simulink model "Crazyflie_Position_controller"  (R2020b)
settings: Solver=VariableStepAuto  StartTime=0.0  StopTime=10.0  RelTol=1e-3
libraries: pid_lib x4
settings Model: Creator=kt012  LastModifiedBy=kt012

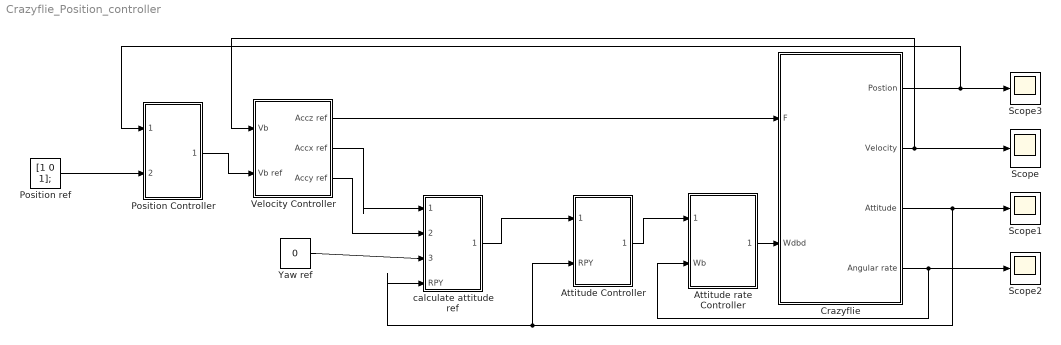
== system Crazyflie_Position_controller ==
  Attitude Controller : Subsystem
  Attitude rate Controller : Subsystem
  Crazyflie : Subsystem
  Position Controller : Subsystem
  Position ref : Constant  Value=[1 0 1];
  Scope{,1..3} (4 alike) : Scope
  Velocity Controller : Subsystem
  Yaw ref : Constant  Value=0
  calculate attitude ref : Subsystem
  wires:
  Crazyflie/1(Postion) -> Position Controller/1(Position), Scope3/1
  Crazyflie/2(Velocity) -> Velocity Controller/1(Vb), Scope/1
  Crazyflie/3(Attitude) -> Attitude Controller/2(RPY), calculate attitude ref/4(RPY), Scope1/1
  Crazyflie/4(Angular rate) -> Attitude rate Controller/2(Wb), Scope2/1
  Attitude rate Controller/1(Wdb_ref) -> Crazyflie/2(Wdbd)
  Attitude Controller/1(Wb_ref) -> Attitude rate Controller/1(Wb_ref)
  Velocity Controller/1(Accz ref) -> Crazyflie/1(F)
  Position Controller/1(Vel ref) -> Velocity Controller/2(Vb ref)
  Velocity Controller/2(Accx ref) -> calculate attitude ref/1(Accel x)
  Velocity Controller/3(Accy ref) -> calculate attitude ref/2("Accel y ")
  Yaw ref/1 -> calculate attitude ref/3(Yaw ref)
  calculate attitude ref/1(Attitude ref) -> Attitude Controller/1(RPY_ref)
  Position ref/1 -> Position Controller/2(Position ref)

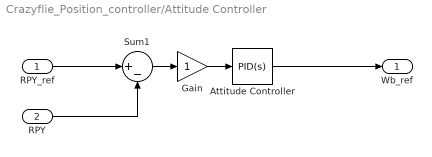
== system Crazyflie_Position_controller/Attitude Controller ==
  RPY_ref : Inport
  RPY : Inport  Port=2
  Attitude Controller : pid_lib/PID Controller  Controller=PID  Form=Parallel  TimeDomain=Continuous-time  UseExternalTs=off  SampleTime=-1  IntegratorMethod=Forward Euler  FilterMethod=Forward Euler  ControllerParametersSource=internal  P=6.0 * 180 / 3.14  I=3.0 * 180 / 3.14  D=25  UseFilter=on  N=100  TunerSelectOption=Transfer Function Based (PID Tuner App)  InitialConditionSource=internal  InitialConditionForIntegrator=0  InitialConditionForFilter=0  DifferentiatorICPrevScaledInput=0  ExternalReset=none  TrackingMode=off  Kt=1  LimitOutput=off  SatLimitsSource=internal  UpperSaturationLimit=inf  LowerSaturationLimit=-inf  LinearizeAsGain=on  AntiWindupMode=none  Kb=1  POutMin=[]  POutMax=[]  IOutMin=[]  IOutMax=[]  DOutMin=[]  DOutMax=[]  NOutMin=[]  NOutMax=[]  SumOutMin=[]  SumOutMax=[]  SaturationOutMin=[]  SaturationOutMax=[]  PParamMin=[]  PParamMax=[]  IParamMin=[]  IParamMax=[]  DParamMin=[]  DParamMax=[]  NParamMin=[]  NParamMax=[]  KbParamMin=[]  KbParamMax=[]  KtParamMin=[]  KtParamMax=[]  KbOutMin=[]  KbOutMax=[]  KtOutMin=[]  KtOutMax=[]  IntegratorOutMin=[]  IntegratorOutMax=[]  FilterOutMin=[]  FilterOutMax=[]  SumI1OutMin=[]  SumI1OutMax=[]  SumI2OutMin=[]  SumI2OutMax=[]  SumI3OutMin=[]  SumI3OutMax=[]  SumI4OutMin=[]  SumI4OutMax=[]  SumDOutMin=[]  SumDOutMax=[]  DifferentiatorOutMin=[]  DifferentiatorOutMax=[]  FilterDiffOutCoefMin=[]  FilterDiffOutCoefMax=[]  ReciprocalOutMin=[]  ReciprocalOutMax=[]  SumDenOutMin=[]  SumDenOutMax=[]  SumNumOutMin=[]  SumNumOutMax=[]  DivideOutMin=[]  DivideOutMax=[]  UdiffTsProdOutMin=[]  UdiffTsProdOutMax=[]  NTsProdOutMin=[]  NTsProdOutMax=[]  UintegralTsProdOutMin=[]  UintegralTsProdOutMax=[]  UngainTsProdOutMin=[]  UngainTsProdOutMax=[]  IntegratorContinuousStateAttributes=''  IntegratorStateMustResolveToSignalObject=off  IntegratorRTWStateStorageClass=Auto  FilterContinuousStateAttributes=''  FilterStateMustResolveToSignalObject=off  FilterRTWStateStorageClass=Auto  ParallelPVariant=InternalParameters  IdealPVariant=Disabled  IVariant=InternalParameters  DVariant=InternalParameters  IntegratorVariant=Continuous  SatVariant=Disabled  AWVariant=Passthrough  PCopyVariant=Disabled  TRVariant=Disabled  FdbkBlocksVariant=Forward  IdealPFdbkVariant=Disabled  SatFdbkVariant=Disabled  DerivativeFilterVariant=ContFilter  NVariant=InternalParameters  NCopyVariant=Disabled  FilterICVariant=InternalICsFilter  IntegratorICVariant=InternalICs  ExternalResetVariant=Disabled  TRSumVariant=Passthrough  SumFdbkVariant=Disabled  SumVariant=Sum_PID  TsampFilterVariant=InternalTs  TsampNgainVariant=Passthrough  TsampIntegralVariant=Passthrough  ExternalSaturationOutDataTypeStr=Inherit: Same as second input
  Gain : Gain
  Sum1 : Sum  Inputs=|+-
  Wb_ref : Outport
  wires:
  Gain/1 -> Attitude Controller/1
  RPY/1 -> Sum1/2
  Sum1/1 -> Gain/1
  Attitude Controller/1 -> Wb_ref/1
  RPY_ref/1 -> Sum1/1

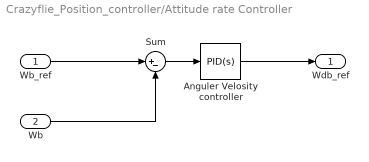
== system Crazyflie_Position_controller/Attitude rate Controller ==
  Wb_ref : Inport
  Wb : Inport  Port=2
  Anguler Velosity controller : pid_lib/PID Controller  Controller=PID  Form=Parallel  TimeDomain=Continuous-time  UseExternalTs=off  SampleTime=-1  IntegratorMethod=Forward Euler  FilterMethod=Forward Euler  ControllerParametersSource=internal  P=250 * 180 / 3.14  I=500 * 180 / 3.14  D=2.5 * 180 / 3.14  UseFilter=on  N=100  TunerSelectOption=Transfer Function Based (PID Tuner App)  InitialConditionSource=internal  InitialConditionForIntegrator=0  InitialConditionForFilter=0  DifferentiatorICPrevScaledInput=0  ExternalReset=none  TrackingMode=off  Kt=1  LimitOutput=off  SatLimitsSource=internal  UpperSaturationLimit=inf  LowerSaturationLimit=-inf  LinearizeAsGain=on  AntiWindupMode=none  Kb=1  POutMin=[]  POutMax=[]  IOutMin=[]  IOutMax=[]  DOutMin=[]  DOutMax=[]  NOutMin=[]  NOutMax=[]  SumOutMin=[]  SumOutMax=[]  SaturationOutMin=[]  SaturationOutMax=[]  PParamMin=[]  PParamMax=[]  IParamMin=[]  IParamMax=[]  DParamMin=[]  DParamMax=[]  NParamMin=[]  NParamMax=[]  KbParamMin=[]  KbParamMax=[]  KtParamMin=[]  KtParamMax=[]  KbOutMin=[]  KbOutMax=[]  KtOutMin=[]  KtOutMax=[]  IntegratorOutMin=[]  IntegratorOutMax=[]  FilterOutMin=[]  FilterOutMax=[]  SumI1OutMin=[]  SumI1OutMax=[]  SumI2OutMin=[]  SumI2OutMax=[]  SumI3OutMin=[]  SumI3OutMax=[]  SumI4OutMin=[]  SumI4OutMax=[]  SumDOutMin=[]  SumDOutMax=[]  DifferentiatorOutMin=[]  DifferentiatorOutMax=[]  FilterDiffOutCoefMin=[]  FilterDiffOutCoefMax=[]  ReciprocalOutMin=[]  ReciprocalOutMax=[]  SumDenOutMin=[]  SumDenOutMax=[]  SumNumOutMin=[]  SumNumOutMax=[]  DivideOutMin=[]  DivideOutMax=[]  UdiffTsProdOutMin=[]  UdiffTsProdOutMax=[]  NTsProdOutMin=[]  NTsProdOutMax=[]  UintegralTsProdOutMin=[]  UintegralTsProdOutMax=[]  UngainTsProdOutMin=[]  UngainTsProdOutMax=[]  IntegratorContinuousStateAttributes=''  IntegratorStateMustResolveToSignalObject=off  IntegratorRTWStateStorageClass=Auto  FilterContinuousStateAttributes=''  FilterStateMustResolveToSignalObject=off  FilterRTWStateStorageClass=Auto  ParallelPVariant=InternalParameters  IdealPVariant=Disabled  IVariant=InternalParameters  DVariant=InternalParameters  IntegratorVariant=Continuous  SatVariant=Disabled  AWVariant=Passthrough  PCopyVariant=Disabled  TRVariant=Disabled  FdbkBlocksVariant=Forward  IdealPFdbkVariant=Disabled  SatFdbkVariant=Disabled  DerivativeFilterVariant=ContFilter  NVariant=InternalParameters  NCopyVariant=Disabled  FilterICVariant=InternalICsFilter  IntegratorICVariant=InternalICs  ExternalResetVariant=Disabled  TRSumVariant=Passthrough  SumFdbkVariant=Disabled  SumVariant=Sum_PID  TsampFilterVariant=InternalTs  TsampNgainVariant=Passthrough  TsampIntegralVariant=Passthrough  ExternalSaturationOutDataTypeStr=Inherit: Same as second input
  Sum : Sum  Inputs=|+-
  Wdb_ref : Outport
  wires:
  Sum/1 -> Anguler Velosity controller/1
  Anguler Velosity controller/1 -> Wdb_ref/1
  Wb/1 -> Sum/2
  Wb_ref/1 -> Sum/1

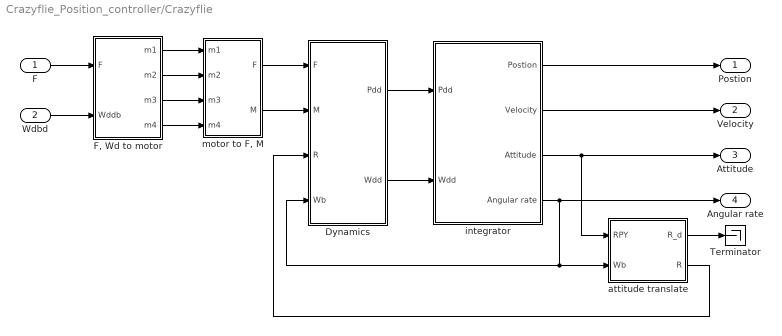
== system Crazyflie_Position_controller/Crazyflie ==
  F : Inport
  Wdbd : Inport  Port=2
  Dynamics : MATLAB Function  TreatAsAtomicUnit=on
  "F, Wd to motor" : MATLAB Function  TreatAsAtomicUnit=on
  Terminator : Terminator
  attitude translate : MATLAB Function  TreatAsAtomicUnit=on
  integrator : Subsystem
  "motor to F, M" : MATLAB Function  TreatAsAtomicUnit=on
  Postion : Outport
  Velocity : Outport  Port=2
  Attitude : Outport  Port=3
  Angular rate : Outport  Port=4
  wires:
  "F, Wd to motor"/1(m1) -> "motor to F, M"/1(m1)
  Wdbd/1 -> "F, Wd to motor"/2(Wddb)
  "F, Wd to motor"/4(m4) -> "motor to F, M"/4(m4)
  "F, Wd to motor"/2(m2) -> "motor to F, M"/2(m2)
  "F, Wd to motor"/3(m3) -> "motor to F, M"/3(m3)
  Dynamics/2(Wdd) -> integrator/2(Wdd)
  "motor to F, M"/2(M) -> Dynamics/2(M)
  integrator/4(Angular rate) -> Angular rate/1, attitude translate/2(Wb), Dynamics/4(Wb)
  "motor to F, M"/1(F) -> Dynamics/1(F)
  F/1 -> "F, Wd to motor"/1(F)
  Dynamics/1(Pdd) -> integrator/1(Pdd)
  integrator/3(Attitude) -> Attitude/1, attitude translate/1(RPY)
  integrator/1(Postion) -> Postion/1
  integrator/2(Velocity) -> Velocity/1
  attitude translate/2(R) -> Dynamics/3(R)
  attitude translate/1(R_d) -> Terminator/1

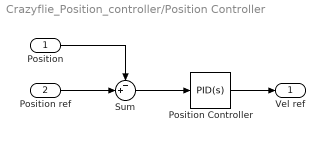
== system Crazyflie_Position_controller/Position Controller ==
  Position : Inport
  Position ref : Inport  Port=2
  Position Controller : pid_lib/PID Controller  Controller=PID  Form=Parallel  TimeDomain=Continuous-time  UseExternalTs=off  SampleTime=-1  IntegratorMethod=Forward Euler  FilterMethod=Forward Euler  ControllerParametersSource=internal  P=2  I=0.5  D=0  UseFilter=on  N=100  TunerSelectOption=Transfer Function Based (PID Tuner App)  InitialConditionSource=internal  InitialConditionForIntegrator=0  InitialConditionForFilter=0  DifferentiatorICPrevScaledInput=0  ExternalReset=none  TrackingMode=off  Kt=1  LimitOutput=off  SatLimitsSource=internal  UpperSaturationLimit=inf  LowerSaturationLimit=-inf  LinearizeAsGain=on  AntiWindupMode=none  Kb=1  POutMin=[]  POutMax=[]  IOutMin=[]  IOutMax=[]  DOutMin=[]  DOutMax=[]  NOutMin=[]  NOutMax=[]  SumOutMin=[]  SumOutMax=[]  SaturationOutMin=[]  SaturationOutMax=[]  PParamMin=[]  PParamMax=[]  IParamMin=[]  IParamMax=[]  DParamMin=[]  DParamMax=[]  NParamMin=[]  NParamMax=[]  KbParamMin=[]  KbParamMax=[]  KtParamMin=[]  KtParamMax=[]  KbOutMin=[]  KbOutMax=[]  KtOutMin=[]  KtOutMax=[]  IntegratorOutMin=[]  IntegratorOutMax=[]  FilterOutMin=[]  FilterOutMax=[]  SumI1OutMin=[]  SumI1OutMax=[]  SumI2OutMin=[]  SumI2OutMax=[]  SumI3OutMin=[]  SumI3OutMax=[]  SumI4OutMin=[]  SumI4OutMax=[]  SumDOutMin=[]  SumDOutMax=[]  DifferentiatorOutMin=[]  DifferentiatorOutMax=[]  FilterDiffOutCoefMin=[]  FilterDiffOutCoefMax=[]  ReciprocalOutMin=[]  ReciprocalOutMax=[]  SumDenOutMin=[]  SumDenOutMax=[]  SumNumOutMin=[]  SumNumOutMax=[]  DivideOutMin=[]  DivideOutMax=[]  UdiffTsProdOutMin=[]  UdiffTsProdOutMax=[]  NTsProdOutMin=[]  NTsProdOutMax=[]  UintegralTsProdOutMin=[]  UintegralTsProdOutMax=[]  UngainTsProdOutMin=[]  UngainTsProdOutMax=[]  IntegratorContinuousStateAttributes=''  IntegratorStateMustResolveToSignalObject=off  IntegratorRTWStateStorageClass=Auto  FilterContinuousStateAttributes=''  FilterStateMustResolveToSignalObject=off  FilterRTWStateStorageClass=Auto  ParallelPVariant=InternalParameters  IdealPVariant=Disabled  IVariant=InternalParameters  DVariant=InternalParameters  IntegratorVariant=Continuous  SatVariant=Disabled  AWVariant=Passthrough  PCopyVariant=Disabled  TRVariant=Disabled  FdbkBlocksVariant=Forward  IdealPFdbkVariant=Disabled  SatFdbkVariant=Disabled  DerivativeFilterVariant=ContFilter  NVariant=InternalParameters  NCopyVariant=Disabled  FilterICVariant=InternalICsFilter  IntegratorICVariant=InternalICs  ExternalResetVariant=Disabled  TRSumVariant=Passthrough  SumFdbkVariant=Disabled  SumVariant=Sum_PID  TsampFilterVariant=InternalTs  TsampNgainVariant=Passthrough  TsampIntegralVariant=Passthrough  ExternalSaturationOutDataTypeStr=Inherit: Same as second input
  Sum : Sum  Inputs=-+|
  Vel ref : Outport
  wires:
  Sum/1 -> Position Controller/1
  Position Controller/1 -> Vel ref/1
  Position ref/1 -> Sum/2
  Position/1 -> Sum/1

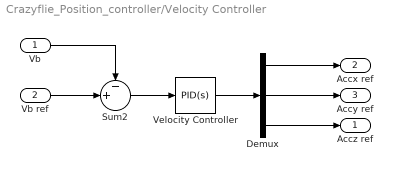
== system Crazyflie_Position_controller/Velocity Controller ==
  Vb : Inport
  Vb ref : Inport  Port=2
  Demux : Demux  Outputs=3
  Sum2 : Sum  Inputs=-+|
  Velocity Controller : pid_lib/PID Controller  Controller=PID  Form=Parallel  TimeDomain=Continuous-time  UseExternalTs=off  SampleTime=-1  IntegratorMethod=Forward Euler  FilterMethod=Forward Euler  ControllerParametersSource=internal  P=25  I=10  D=0  UseFilter=on  N=100  TunerSelectOption=Transfer Function Based (PID Tuner App)  InitialConditionSource=internal  InitialConditionForIntegrator=0  InitialConditionForFilter=0  DifferentiatorICPrevScaledInput=0  ExternalReset=none  TrackingMode=off  Kt=1  LimitOutput=off  SatLimitsSource=internal  UpperSaturationLimit=inf  LowerSaturationLimit=-inf  LinearizeAsGain=on  AntiWindupMode=none  Kb=1  POutMin=[]  POutMax=[]  IOutMin=[]  IOutMax=[]  DOutMin=[]  DOutMax=[]  NOutMin=[]  NOutMax=[]  SumOutMin=[]  SumOutMax=[]  SaturationOutMin=[]  SaturationOutMax=[]  PParamMin=[]  PParamMax=[]  IParamMin=[]  IParamMax=[]  DParamMin=[]  DParamMax=[]  NParamMin=[]  NParamMax=[]  KbParamMin=[]  KbParamMax=[]  KtParamMin=[]  KtParamMax=[]  KbOutMin=[]  KbOutMax=[]  KtOutMin=[]  KtOutMax=[]  IntegratorOutMin=[]  IntegratorOutMax=[]  FilterOutMin=[]  FilterOutMax=[]  SumI1OutMin=[]  SumI1OutMax=[]  SumI2OutMin=[]  SumI2OutMax=[]  SumI3OutMin=[]  SumI3OutMax=[]  SumI4OutMin=[]  SumI4OutMax=[]  SumDOutMin=[]  SumDOutMax=[]  DifferentiatorOutMin=[]  DifferentiatorOutMax=[]  FilterDiffOutCoefMin=[]  FilterDiffOutCoefMax=[]  ReciprocalOutMin=[]  ReciprocalOutMax=[]  SumDenOutMin=[]  SumDenOutMax=[]  SumNumOutMin=[]  SumNumOutMax=[]  DivideOutMin=[]  DivideOutMax=[]  UdiffTsProdOutMin=[]  UdiffTsProdOutMax=[]  NTsProdOutMin=[]  NTsProdOutMax=[]  UintegralTsProdOutMin=[]  UintegralTsProdOutMax=[]  UngainTsProdOutMin=[]  UngainTsProdOutMax=[]  IntegratorContinuousStateAttributes=''  IntegratorStateMustResolveToSignalObject=off  IntegratorRTWStateStorageClass=Auto  FilterContinuousStateAttributes=''  FilterStateMustResolveToSignalObject=off  FilterRTWStateStorageClass=Auto  ParallelPVariant=InternalParameters  IdealPVariant=Disabled  IVariant=InternalParameters  DVariant=InternalParameters  IntegratorVariant=Continuous  SatVariant=Disabled  AWVariant=Passthrough  PCopyVariant=Disabled  TRVariant=Disabled  FdbkBlocksVariant=Forward  IdealPFdbkVariant=Disabled  SatFdbkVariant=Disabled  DerivativeFilterVariant=ContFilter  NVariant=InternalParameters  NCopyVariant=Disabled  FilterICVariant=InternalICsFilter  IntegratorICVariant=InternalICs  ExternalResetVariant=Disabled  TRSumVariant=Passthrough  SumFdbkVariant=Disabled  SumVariant=Sum_PID  TsampFilterVariant=InternalTs  TsampNgainVariant=Passthrough  TsampIntegralVariant=Passthrough  ExternalSaturationOutDataTypeStr=Inherit: Same as second input
  Accz ref : Outport
  Accx ref : Outport  Port=2
  Accy ref : Outport  Port=3
  wires:
  Demux/2 -> Accy ref/1
  Velocity Controller/1 -> Demux/1
  Sum2/1 -> Velocity Controller/1
  Demux/1 -> Accx ref/1
  Vb/1 -> Sum2/1
  Demux/3 -> Accz ref/1
  Vb ref/1 -> Sum2/2

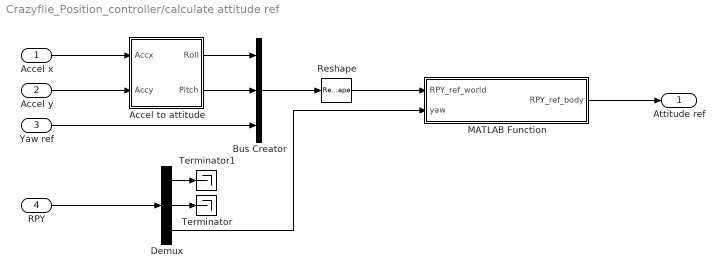
== system Crazyflie_Position_controller/calculate attitude ref ==
  Accel x : Inport
  "Accel y " : Inport  Port=2
  Yaw ref : Inport  Port=3
  RPY : Inport  Port=4
  Accel to attitude : MATLAB Function  TreatAsAtomicUnit=on
  Bus Creator : BusCreator  Inputs=3
  Demux : Demux  Outputs=3
  MATLAB Function : MATLAB Function  TreatAsAtomicUnit=on
  Reshape : Reshape  OutputDimensionality=Row vector (2-D)
  Terminator : Terminator
  Terminator1 : Terminator
  Attitude ref : Outport
  wires:
  Accel x/1 -> Accel to attitude/1(Accx)
  Accel to attitude/1(Roll) -> Bus Creator/1
  "Accel y "/1 -> Accel to attitude/2(Accy)
  Accel to attitude/2(Pitch) -> Bus Creator/2
  Yaw ref/1 -> Bus Creator/3
  MATLAB Function/1(RPY_ref_body) -> Attitude ref/1
  RPY/1 -> Demux/1
  Demux/3 -> MATLAB Function/2(yaw)
  Demux/2 -> Terminator/1
  Demux/1 -> Terminator1/1
  Reshape/1 -> MATLAB Function/1(RPY_ref_world)
  Bus Creator/1 -> Reshape/1

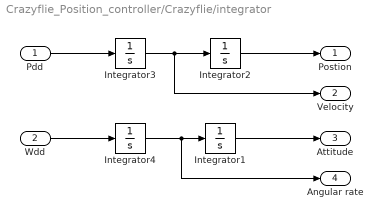
== system Crazyflie_Position_controller/Crazyflie/integrator ==
  Pdd : Inport
  Wdd : Inport  Port=2
  Integrator1 : Integrator  InitialCondition=[0 0 1];
  Integrator2 : Integrator  InitialCondition=[0 0 0];
  Integrator3 : Integrator  InitialCondition=[0 0 0];
  Integrator4 : Integrator  InitialCondition=[0 0 0];
  Postion : Outport
  Velocity : Outport  Port=2
  Attitude : Outport  Port=3
  Angular rate : Outport  Port=4
  wires:
  Wdd/1 -> Integrator4/1
  Integrator4/1 -> Angular rate/1, Integrator1/1
  Integrator1/1 -> Attitude/1
  Pdd/1 -> Integrator3/1
  Integrator3/1 -> Integrator2/1, Velocity/1
  Integrator2/1 -> Postion/1

== matlab function Crazyflie_Position_controller/Crazyflie/F, Wd to motor ==
  data: F input; Wddb input; m1 output; m2 output; m3 output; m4 output
 function [m1, m2, m3, m4]= fcn(F, Wddb)

% F [16bit] Wddb [16bit]
F = F * 1000 + 32000;

r = min(max(-32000, Wddb(1)), 32000)/2;
p = min(max(-32000, Wddb(2)), 32000)/2;
y = min(max(-32000, Wddb(3)), 32000);

m1 = min(max(0,F - r - p + y), 2^16);
m2 = min(max(0,F - r + p - y), 2^16);
m3 = min(max(0,F + r + p + y), 2^16);
m4 = min(max(0,F + r - p - y), 2^16);

% formation +
% r = min(max(-32000, Wddb(1)), 32000);
% p = min(max(-32000, Wddb(2)), 32000);
% y = min(max(-32000, Wddb(3)), 32000);
% m1 = min(max(0, + p + y), 2^16);
% m2 = min(max(0, - r - y), 2^16);
% m3 = min(max(0, - p + y), 2^16);
% m4 = min(max(0, + r - y), 2^16);

%         ^y
%         |
%         |
%   m3          m4
%
%                    ------>x
%
%   m2          m1

== matlab function Crazyflie_Position_controller/Crazyflie/attitude translate ==
  data: RPY input; Wb input; R_d output; R output
function [R_d, R]= fcn(RPY, Wb)
% 角速度 Vee演算
Wb = [ 0     -Wb(3)   Wb(2);
       Wb(3)  0       -Wb(1);
      -Wb(2)  Wb(1)   0   ];

% RPYから回転行列計算
roll = RPY(1);
pitch= RPY(2);
yaw = RPY(3);

R3 = [ cos(yaw) -sin(yaw) 0; sin(yaw) cos(yaw) 0; 0 0 1];              % ヨー角
R2 = [ cos(pitch) 0 -sin(pitch); 0 1 0; sin(pitch) 0 cos(pitch) ];     % ピッチ角
R1 = [ 1 0 0; 0 cos(roll) -sin(roll); 0 sin(roll) cos(roll)];          % ロール角

R = R1 * R2 * R3;   % 回転行列（ボディー　-> ワールド）

R_d = R * Wb;       % 微小時間の回転行列

== matlab function Crazyflie_Position_controller/calculate attitude ref/Accel to attitude ==
  data: Accx input; Roll output; Pitch output; Accy input
function [Roll, Pitch]= fcn(Accx, Accy)

Roll = -Accy * 3.14 / 180;
Pitch = -Accx* 3.14 / 180;

== matlab function Crazyflie_Position_controller/Crazyflie/motor to F, M ==
  data: F output; m1 input; m2 input; M output; m3 input; m4 input
function [F, M] = func(m1, m2, m3, m4)

% F [16bit] Wddb [16bit]

Armlength = 0.092/2;
m1 = 2.130295 * 10^(-11) * m1^2 + 1.032633 * 10^(-6) * m1 + 5.484560 * 10^(-4);
m2 = 2.130295 * 10^(-11) * m2^2 + 1.032633 * 10^(-6) * m2 + 5.484560 * 10^(-4);
m3 = 2.130295 * 10^(-11) * m3^2 + 1.032633 * 10^(-6) * m3 + 5.484560 * 10^(-4);
m4 = 2.130295 * 10^(-11) * m4^2 + 1.032633 * 10^(-6) * m4 + 5.484560 * 10^(-4);

% calculate thrust
F = m1 + m2 + m3 + m4;

% calculate moment formation X
M1 = Armlength / sqrt(2) * (m3 + m4 - m1 - m2);
M2 = -Armlength / sqrt(2) * (-m3 - m2 + m1 + m4);

% calculate moment formation + 
% M1 = Armlength  * (m4 - m2);
% M2 = Armlength * (m1 - m3);

M3 = m1 + m3 - m2 - m4;

M = [M1 M2 M3]';

== matlab function Crazyflie_Position_controller/Crazyflie/Dynamics ==
  data: Pdd output; F input; M input; R input; Wb input; Wdd output
function [Pdd,Wdd] = fcn(F, M, R, Wb)
m = 0.028;
e3 = [0 0 1]';
g = 9.8;
% % crazyflie
I = [16.571710 0.830806 0.718277;
     0.830806 16.655602 1.800197;
     0.718277 1.800197 29.261652] * 10^(-6);      % crazyflieの慣性モーメント（kg・m^2）
% I = [1 0 0;
%      0 1 0;
%      0 0 1] * 10^(-6);
% 機体上向き加速度
Pdd = (R*F*e3 - m*g*e3)/m;

% 各加速度計算（ボディー座標系）
Wdd = pinv(I)*(M - cross(Wb, I * Wb));

== matlab function Crazyflie_Position_controller/calculate attitude ref/MATLAB Function ==
  data: RPY_ref_world input; RPY_ref_body output; yaw input
function RPY_ref_body = fcn(RPY_ref_world, yaw)

Ryaw = [cos(yaw) -sin(yaw) 0;
        sin(yaw)  cos(yaw) 0;
        0         0        1];
tmp = Ryaw' * RPY_ref_world';
RPY_ref_body = [tmp(1) tmp(2) tmp(3)];
